simulink model "sim_EKF"  (R2018a)
settings: Solver=FixedStepAuto  StartTime=0.0  StopTime=50  FixedStep=dT  RelTol=1e-3
values from neighbouring files (symbols this model uses):
  beta = 8/3    (= 2.66666666667)    [scr_EKF.m]
  dT = 0.01    [scr_EKF.m]    (also in starshot_ACS_setup.m = 0.1)
  Hd = H    [scr_EKF.m]    (also in starshot_ACS_setup.m)
  k_noise = 1    [scr_EKF.m]    (also in starshot_ACS_setup.m = 3e-05)
  Q = [100,  0,  0 ... (first row only)    [scr_EKF.m]    (also in starshot_ACS_setup.m = 0.02*diag([0.008,0.07,0.005,0.1,0.1,0.1]))
  Rd = (1/dT)*R    [scr_EKF.m]    (also in starshot_ACS_setup.m = Rn)
  rho = 28    [scr_EKF.m]
  sigma = 10    [scr_EKF.m]
libraries: simulink x3
settings Model: Creator=Hakan  LastModifiedBy=Hakan

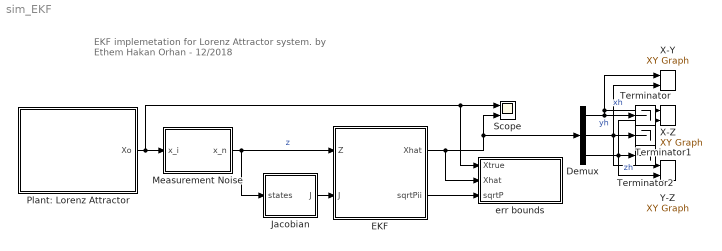
== system sim_EKF ==
  note: EKF implemetation for Lorenz Attractor system.
      | by Ethem Hakan Orhan - 12/2018
  Demux : Demux  Outputs=3
  EKF : Subsystem
  Jacobian : MATLAB Function  TreatAsAtomicUnit=on
  Measurement Noise : Subsystem
  Plant: Lorenz Attractor : Subsystem
  Scope : Scope  NumInputPorts=2
  Terminator : Terminator
  Terminator1 : Terminator
  Terminator2 : Terminator
  X-Y : simulink/Sinks/XY Graph  xmin=-30  xmax=30  ymin=-30  ymax=30  st=-1
  X-Z : simulink/Sinks/XY Graph  xmin=-30  xmax=30  ymin=0  ymax=50  st=-1
  Y-Z : simulink/Sinks/XY Graph  xmin=-30  xmax=30  ymin=0  ymax=50  st=-1
  err bounds : Subsystem
  wires:
  Jacobian/1(J) -> EKF/2(J)
  EKF/1(Xhat) -> err bounds/2(Xhat), Demux/1, Scope/2
  Measurement Noise/1(x_n) -> EKF/1(Z), Jacobian/1(states)  "z"
  Demux/1 -> X-Y/1, X-Z/1, Terminator/1  "xh"
  Demux/2 -> X-Y/2, Y-Z/1, Terminator1/1  "yh"
  Demux/3 -> Y-Z/2, X-Z/2, Terminator2/1  "zh"
  Plant: Lorenz Attractor/1(Xo) -> err bounds/1(Xtrue), Scope/1, Measurement Noise/1(x_i)
  EKF/2(sqrtPii) -> err bounds/3(sqrtP)

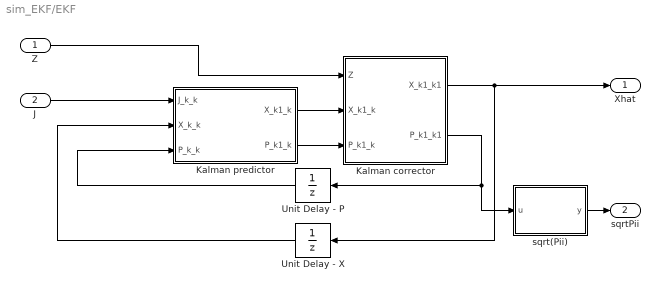
== system sim_EKF/EKF ==
  Z : Inport
  J : Inport  Port=2
  Kalman corrector : MATLAB Function  TreatAsAtomicUnit=on
  Kalman predictor : MATLAB Function  TreatAsAtomicUnit=on
  Unit Delay - P : UnitDelay  InitialCondition=eye(3)  SampleTime=-1
  Unit Delay - X : UnitDelay  InitialCondition=[0 0 0]'  SampleTime=-1
  sqrt(Pii) : MATLAB Function  TreatAsAtomicUnit=on
  Xhat : Outport
  sqrtPii : Outport  Port=2
  wires:
  Unit Delay - P/1 -> Kalman predictor/3(P_k_k)
  J/1 -> Kalman predictor/1(J_k_k)
  Kalman corrector/2(P_k1_k1) -> sqrt(Pii)/1(u), Unit Delay - P/1
  Kalman corrector/1(X_k1_k1) -> Xhat/1, Unit Delay - X/1
  sqrt(Pii)/1(y) -> sqrtPii/1
  Kalman predictor/1(X_k1_k) -> Kalman corrector/2(X_k1_k)
  Kalman predictor/2(P_k1_k) -> Kalman corrector/3(P_k1_k)
  Unit Delay - X/1 -> Kalman predictor/2(X_k_k)
  Z/1 -> Kalman corrector/1(Z)

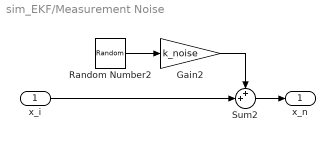
== system sim_EKF/Measurement Noise ==
  x_i : Inport
  Gain2 : Gain  Gain=k_noise
  Random Number2 : RandomNumber  Variance=0.15  Seed=[4,5,6]  SampleTime=dT
  Sum2 : Sum  Inputs=++|
  x_n : Outport
  wires:
  Random Number2/1 -> Gain2/1
  Gain2/1 -> Sum2/1
  x_i/1 -> Sum2/2
  Sum2/1 -> x_n/1

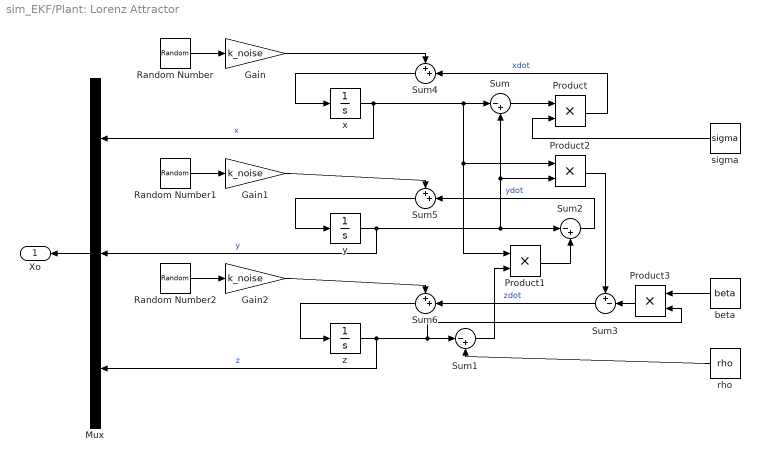
== system sim_EKF/Plant: Lorenz Attractor ==
  Gain : Gain  Gain=k_noise
  Gain1 : Gain  Gain=k_noise
  Gain2 : Gain  Gain=k_noise
  Mux : Mux  Inputs=3
  Product{,1..3} (4 alike) : Product  Inputs=**
  Random Number : RandomNumber  Variance=0.1  Seed=1  SampleTime=dT
  Random Number1 : RandomNumber  Variance=0.1  Seed=2  SampleTime=dT
  Random Number2 : RandomNumber  Variance=0.1  Seed=3  SampleTime=dT
  Sum : Sum  Inputs=|-+
  Sum1 : Sum  Inputs=|-+
  Sum2 : Sum  Inputs=|-+
  Sum3 : Sum  Inputs=+-|
  Sum4 : Sum  Inputs=++|
  Sum5 : Sum  Inputs=++|
  Sum6 : Sum  Inputs=++|
  beta : Constant  Value=beta
  rho : Constant  Value=rho
  sigma : Constant  Value=sigma
  x : Integrator  InitialCondition=1
  y : Integrator  InitialCondition=1
  z : Integrator  InitialCondition=1
  Xo : Outport
  wires:
  z/1 -> Mux/3, Product3/2, Sum1/1  "z"
  sigma/1 -> Product/2
  Product1/1 -> Sum2/2
  y/1 -> Mux/2, Sum/2, Product2/2, Sum2/1  "y"
  rho/1 -> Sum1/2
  x/1 -> Mux/1, Product1/1, Product2/1, Sum/1  "x"
  Sum/1 -> Product/1
  Sum1/1 -> Product1/2
  Product3/1 -> Sum3/2
  beta/1 -> Product3/1
  Product2/1 -> Sum3/1
  Product/1 -> Sum4/2  "xdot"
  Sum4/1 -> x/1
  Random Number/1 -> Gain/1
  Gain/1 -> Sum4/1
  Sum2/1 -> Sum5/2  "ydot"
  Sum5/1 -> y/1
  Random Number1/1 -> Gain1/1
  Random Number2/1 -> Gain2/1
  Gain1/1 -> Sum5/1
  Sum3/1 -> Sum6/2  "zdot"
  Sum6/1 -> z/1
  Gain2/1 -> Sum6/1
  Mux/1 -> Xo/1

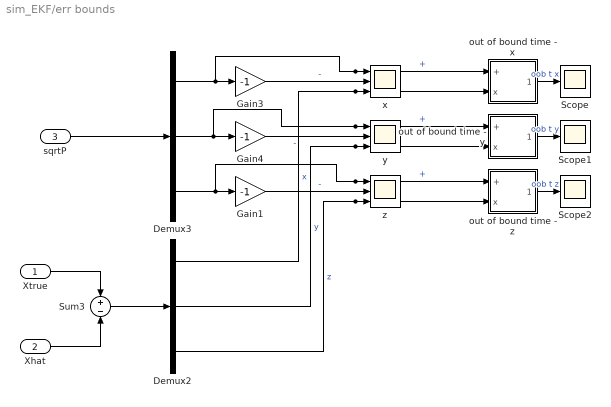
== system sim_EKF/err bounds ==
  Xtrue : Inport
  Xhat : Inport  Port=2
  sqrtP : Inport  Port=3
  Demux2 : Demux  Outputs=3
  Demux3 : Demux  Outputs=3
  Gain1 : Gain  Gain=-1
  Gain3 : Gain  Gain=-1
  Gain4 : Gain  Gain=-1
  Scope : Scope
  Scope1 : Scope
  Scope2 : Scope
  Sum3 : Sum  Inputs=+-
  out of bound time - x : Subsystem
  out of bound time - y : Subsystem
  out of bound time - z : Subsystem
  x : Scope  NumInputPorts=3
  y : Scope  NumInputPorts=3
  z : Scope  NumInputPorts=3
  wires:
  sqrtP/1 -> Demux3/1
  Xhat/1 -> Sum3/2
  Xtrue/1 -> Sum3/1
  Sum3/1 -> Demux2/1
  Demux3/2 -> Gain4/1, out of bound time - y/1(+), y/1  "+"
  Demux3/1 -> Gain3/1, out of bound time - x/1(+), x/1  "+"
  Demux2/1 -> out of bound time - x/2(x), x/3  "x"
  Gain4/1 -> y/2  "-"
  Gain3/1 -> x/2  "-"
  Demux2/2 -> out of bound time - y/2(x), y/3  "y"
  Demux3/3 -> out of bound time - z/1(+), z/1, Gain1/1  "+"
  Gain1/1 -> z/2  "-"
  Demux2/3 -> out of bound time - z/2(x), z/3  "z"
  out of bound time - x/1(clock_o) -> Scope/1  "oob t x"
  out of bound time - y/1(clock_o) -> Scope1/1  "oob t y"
  out of bound time - z/1(clock_o) -> Scope2/1  "oob t z"

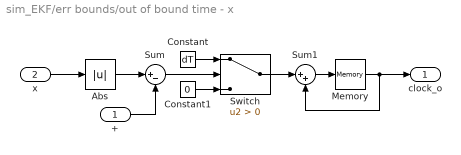
== system sim_EKF/err bounds/out of bound time - x ==
  + : Inport
  x : Inport  Port=2
  Abs : Abs
  Constant : Constant  Value=dT
  Constant1 : Constant  Value=0
  Memory : Memory
  Sum : Sum  Inputs=|+-
  Sum1 : Sum  Inputs=|++
  Switch : Switch  Criteria=u2 > Threshold
  clock_o : Outport
  wires:
  Memory/1 -> clock_o/1, Sum1/2
  Sum1/1 -> Memory/1
  +/1 -> Sum/2
  x/1 -> Abs/1
  Abs/1 -> Sum/1
  Sum/1 -> Switch/2
  Constant/1 -> Switch/1
  Constant1/1 -> Switch/3
  Switch/1 -> Sum1/1

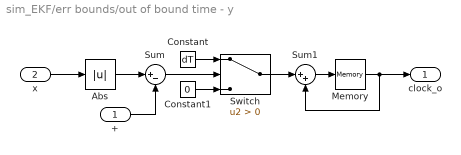
== system sim_EKF/err bounds/out of bound time - y ==
  + : Inport
  x : Inport  Port=2
  Abs : Abs
  Constant : Constant  Value=dT
  Constant1 : Constant  Value=0
  Memory : Memory
  Sum : Sum  Inputs=|+-
  Sum1 : Sum  Inputs=|++
  Switch : Switch  Criteria=u2 > Threshold
  clock_o : Outport
  wires:
  Memory/1 -> clock_o/1, Sum1/2
  Sum1/1 -> Memory/1
  +/1 -> Sum/2
  x/1 -> Abs/1
  Abs/1 -> Sum/1
  Sum/1 -> Switch/2
  Constant/1 -> Switch/1
  Constant1/1 -> Switch/3
  Switch/1 -> Sum1/1

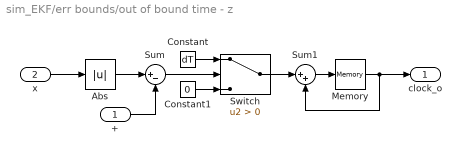
== system sim_EKF/err bounds/out of bound time - z ==
  + : Inport
  x : Inport  Port=2
  Abs : Abs
  Constant : Constant  Value=dT
  Constant1 : Constant  Value=0
  Memory : Memory
  Sum : Sum  Inputs=|+-
  Sum1 : Sum  Inputs=|++
  Switch : Switch  Criteria=u2 > Threshold
  clock_o : Outport
  wires:
  Memory/1 -> clock_o/1, Sum1/2
  Sum1/1 -> Memory/1
  +/1 -> Sum/2
  x/1 -> Abs/1
  Abs/1 -> Sum/1
  Sum/1 -> Switch/2
  Constant/1 -> Switch/1
  Constant1/1 -> Switch/3
  Switch/1 -> Sum1/1

== matlab function sim_EKF/EKF/Kalman corrector ==
  data: Z input; X_k1_k1 output; X_k1_k input; P_k1_k input; P_k1_k1 output; Hd parameter; Rd parameter
function [X_k1_k1, P_k1_k1] = fcn(Z, X_k1_k, P_k1_k, Hd, Rd)

K_k1 = P_k1_k * Hd' * inv(Hd*P_k1_k*Hd' + Rd);
P_k1_k1 = P_k1_k - K_k1*(Hd*P_k1_k*Hd' + Rd)*K_k1';
X_k1_k1 = X_k1_k + K_k1* (Z - Hd*X_k1_k);

== matlab function sim_EKF/Jacobian ==
  data: states input; J output; rho parameter; sigma parameter; beta parameter
function J = fcn(states, rho, sigma, beta)

x = states(1);
y = states(2);
z = states(3);

J = [-sigma, sigma,  0; ...
     rho-z,   -1,   -x; ...
      y,       x,  -beta];

== matlab function sim_EKF/EKF/Kalman predictor ==
  data: J_k_k input; X_k1_k output; X_k_k input; P_k_k input; P_k1_k output; dT parameter; Q parameter
function [X_k1_k, P_k1_k] = fcn(J_k_k, X_k_k, P_k_k, dT, Q)

A = J_k_k;

Ad = expm(A*dT);

F = [-A, Q; zeros(3), A'];
G = expm(F*dT);

Gur = G(1:3, 4:6);
Glr = G(4:6, 4:6);

Qd = Glr'*Gur;

X_k1_k = Ad*X_k_k; 
P_k1_k = Ad*P_k_k*Ad' + Qd;

== matlab function sim_EKF/EKF/sqrt(Pii) ==
  data: u input; y output
function y = fcn(u)

y = sqrt(diag(u));
